simulink model "arm_sim"  (R2015a)
settings: Solver=ode45  StartTime=0.0  StopTime=200  RelTol=1e-3
InitFcn:
  | param
undefined symbols (not defined in the file or in its folder): arm_ctrl, drawArm, P
settings Model: Creator=beard  LastModifiedBy=beard
settings DataIOCC: SignalLoggingSaveFormat=ModelDataLogs
settings OptimizationCC: ExpressionDepthLimit=2147483647  InitFltsAndDblsToZero=on
settings DebuggingCC: UnderspecifiedInitializationDetection=Classic  MergeDetectMultiDrivingBlocksExec=none  SolverPrmCheckMsg=warning  FcnCallInpInsideContextMsg=UseLocalSettings  StateNameClashWarn=warning
settings GRTTargetCC: CombineOutputUpdateFcns=off  GRTInterface=on

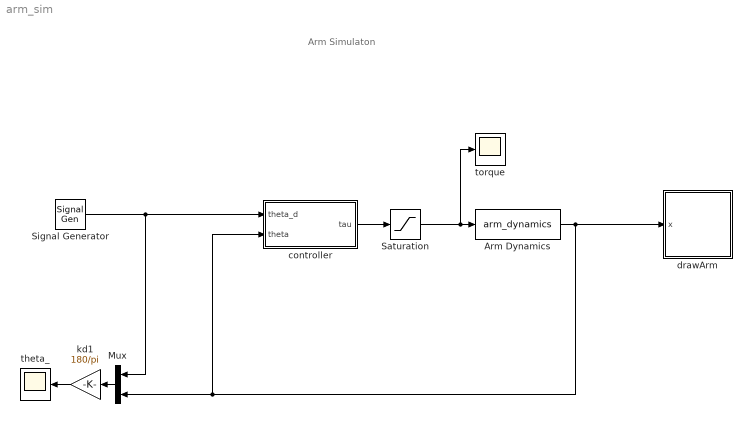
== system arm_sim ==
  note: Arm Simulaton
  Arm Dynamics : S-Function  FunctionName=arm_dynamics  Parameters=AP
  Mux : Mux  Inputs=2
  Saturation : Saturate  UpperLimit=P.tau_max  LowerLimit=-P.tau_max
  Signal Generator : SignalGenerator  WaveForm=square  Amplitude=25*pi/180  Frequency=.05
  controller : Subsystem
  drawArm : Subsystem
      mask Display: image(imread('tv.jpg'))
  kd1 : Gain  Gain=180/pi
  theta_ : Scope
      settings: TimeRange=40  YMin=-27.5  YMax=27.5
  torque : Scope
      settings: YMin=0.15  YMax=1
  wires:
  Signal Generator/1 -> Mux/1, controller/1(theta_d)
  Arm Dynamics/1 -> controller/2(theta), Mux/2, drawArm/1(x)
  Mux/1 -> kd1/1
  kd1/1 -> theta_/1
  Saturation/1 -> Arm Dynamics/1, torque/1
  controller/1(tau) -> Saturation/1

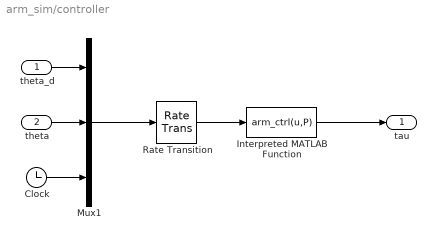
== system arm_sim/controller ==
  theta_d : Inport
  theta : Inport  Port=2
  Clock : Clock
  Interpreted MATLAB Function : MATLABFcn  MATLABFcn=arm_ctrl(u,P)  OutputDimensions=1
  Mux1 : Mux  Inputs=3
  Rate Transition : RateTransition  OutPortSampleTime=P.Ts
  tau : Outport
  wires:
  Mux1/1 -> Rate Transition/1
  theta_d/1 -> Mux1/1
  theta/1 -> Mux1/2
  Interpreted MATLAB Function/1 -> tau/1
  Clock/1 -> Mux1/3
  Rate Transition/1 -> Interpreted MATLAB Function/1

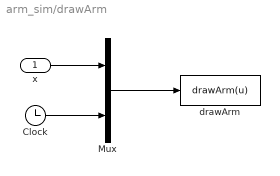
== system arm_sim/drawArm ==
  x : Inport
  Clock : Clock
  Mux : Mux  Inputs=2
  drawArm : MATLABFcn  MATLABFcn=drawArm(u)  OutputDimensions=0  SampleTime=0.1
  wires:
  Mux/1 -> drawArm/1
  x/1 -> Mux/1
  Clock/1 -> Mux/2
